simulink model "problem9"  (R2020b)
settings: Solver=ode23tb  StartTime=0.0  StopTime=1  MaxStep=Ts  RelTol=1e-3  EnableMultiTasking=on
InitFcn:
  | Ts=10e-6;
settings Model: Creator=srikanth  LastModifiedBy=Makrand Raut Dessai
settings DataIOCC: LimitDataPoints=on  SaveFormat=Array  SignalLoggingSaveFormat=ModelDataLogs  ReturnWorkspaceOutputs=off
settings OptimizationCC: ExpressionDepthLimit=2147483647  LifeSpan=inf
settings DebuggingCC: UnderspecifiedInitializationDetection=Classic  MergeDetectMultiDrivingBlocksExec=none  SolverPrmCheckMsg=warning  FcnCallInpInsideContextMsg=warning  StateNameClashWarn=warning  SFUnexpectedBacktrackingDiag=warning  SFNoUnconditionalDefaultTransitionDiag=warning  SFExecutionAtInitializationDiag=none  ArithmeticOperatorsInVariantConditions=warning
settings HardwareCC: ProdBitPerPointer=32  ProdBitPerSizeT=32  ProdBitPerPtrDiffT=32  ProdLargestAtomicFloat=None  ProdIntDivRoundTo=Undefined  ProdEndianess=Unspecified  ProdWordSize=32  ProdHWDeviceType=32-bit Generic
settings ModelReferenceCC: PropagateSignalLabelsOutOfModel=off
settings SFSimCC: SimUseLocalCustomCode=off  CustomCodeUndefinedFunction=UseInterfaceOnly
settings RTWCC: RTWUseLocalCustomCode=off
settings CodeAppCC: StateflowObjectComments=on
settings GRTTargetCC: TargetLangStandard=C89/C90 (ANSI)  CombineOutputUpdateFcns=off  GRTInterface=on
settings ConfigComp: CovMetricSettings=dw  CovSaveCumulativeToWorkspaceVar=on  CovSaveSingleToWorkspaceVar=on  CovExternalEMLEnable=off

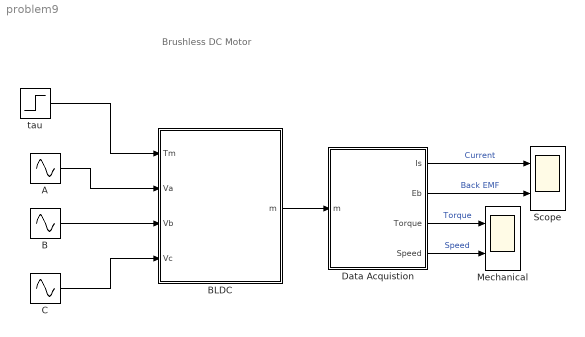
== system problem9 ==
  note: Brushless DC Motor
  A : Sin  Amplitude=220*sqrt(2)  Frequency=2*pi*50  SampleTime=Ts
  B : Sin  Amplitude=220*sqrt(2)  Frequency=2*pi*50  Phase=-2*pi/3  SampleTime=Ts
  BLDC : Subsystem  mask(Brushless DC Motor :){Rs=1.43, Ls=9.4e-3, flux=0.2158, J=1.5e-3, B=2e-3, p=4}
      mask prompts: Rs "Resistance - Rs [ohms] :"; Ls "Inductance - Ls [H] :"; flux "Flux - [wb]"; J "Rotor Inertia - J [kg-m^2]"; B "Friction Coefficient - B :"; p "No: poles of Motor :"
      mask help: Brushless DC Motor inducing trapezoidal Back EMF
      mask init:
      | trap=0.5;
      mask Display: fprintf('BLDC')
  C : Sin  Amplitude=220*sqrt(2)  Frequency=2*pi*50  Phase=2*pi/3  SampleTime=Ts
  Data Acquistion : Subsystem
  Mechanical : Scope  NumInputPorts=2
  Scope : Scope  NumInputPorts=2
  tau : Step  Time=0.5  After=10  SampleTime=0
  wires:
  BLDC/1(m) -> Data Acquistion/1(m)
  Data Acquistion/1(Is) -> Scope/1  "Current"
  Data Acquistion/2(Eb) -> Scope/2  "Back EMF"
  Data Acquistion/3(Torque) -> Mechanical/1  "Torque"
  Data Acquistion/4(Speed) -> Mechanical/2  "Speed"
  tau/1 -> BLDC/1(Tm)
  A/1 -> BLDC/2(Va)
  B/1 -> BLDC/3(Vb)
  C/1 -> BLDC/4(Vc)

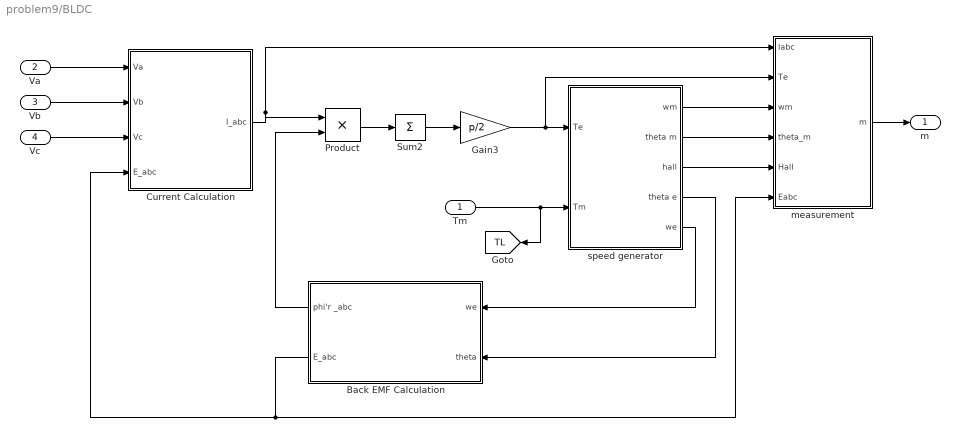
== system problem9/BLDC ==
  Tm : Inport
  Va : Inport  Port=2
  Vb : Inport  Port=3
  Vc : Inport  Port=4
  Back EMF Calculation : Subsystem
  Current Calculation : Subsystem
  Gain3 : Gain  Gain=p/2  SaturateOnIntegerOverflow=on  OutDataTypeStr=Inherit: Same as input  ParamDataTypeStr=Inherit: Same as input
  Product : Product  SaturateOnIntegerOverflow=on  OutDataTypeStr=Inherit: Same as first input
  Sum2 : Sum  Inputs=+  SaturateOnIntegerOverflow=on
  measurement : Subsystem
  speed generator : Subsystem
  m : Outport
  tag scope: TL=global
  wires:
  Vc/1 -> Current Calculation/3(Vc)
  Vb/1 -> Current Calculation/2(Vb)
  Va/1 -> Current Calculation/1(Va)
  measurement/1(m) -> m/1
  speed generator/4(theta e) -> Back EMF Calculation/2(theta)
  speed generator/3(hall) -> measurement/5(Hall)
  speed generator/2(theta m) -> measurement/4(theta_m)
  speed generator/1(wm) -> measurement/3(wm)
  Tm/1 -> [TL], speed generator/2(Tm)
  Back EMF Calculation/1(phi'r _abc) -> Product/2
  Product/1 -> Sum2/1
  Sum2/1 -> Gain3/1
  Gain3/1 -> measurement/2(Te), speed generator/1(Te)
  speed generator/5(we) -> Back EMF Calculation/1(we)
  Back EMF Calculation/2(E_abc) -> Current Calculation/4(E_abc), measurement/6(Eabc)
  Current Calculation/1(I_abc) -> Product/1, measurement/1(Iabc)

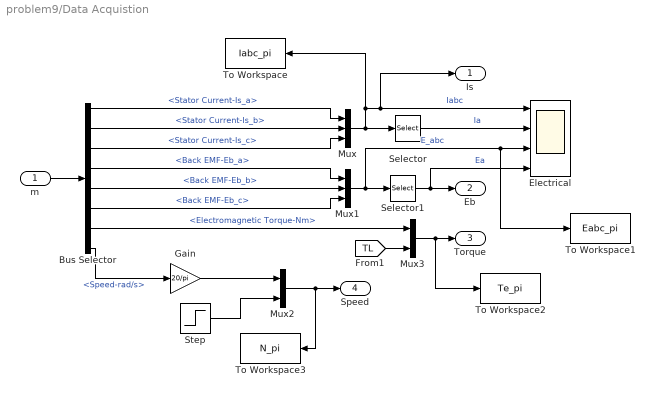
== system problem9/Data Acquistion ==
  m : Inport
  Bus Selector : BusSelector  OutputSignals=Stator Current-Is_a,Stator Current-Is_b,Stator Current-Is_c,Back EMF-Eb_a,Back EMF-Eb_b,Back EMF-Eb_c,Electromagnetic Torque-Nm,Speed-rad/s
  Electrical : Scope  NumInputPorts=4
  Gain : Gain  Gain=20/pi
  Mux : Mux  Inputs=3
  Mux1 : Mux  Inputs=3
  Mux2 : Mux  Inputs=2
  Mux3 : Mux  Inputs=2
  Selector : Selector  InputPortWidth=3  IndexOptions=Index vector (dialog)  Indices=[1 ]  OutputSizes=1
  Selector1 : Selector  InputPortWidth=3  IndexOptions=Index vector (dialog)  Indices=[1 ]  OutputSizes=1
  Step : Step  After=3000  SampleTime=0
  To Workspace : ToWorkspace  VariableName=Iabc_pi  SampleTime=Ts
  To Workspace1 : ToWorkspace  VariableName=Eabc_pi  SampleTime=Ts
  To Workspace2 : ToWorkspace  VariableName=Te_pi  SampleTime=Ts
  To Workspace3 : ToWorkspace  VariableName=N_pi  SampleTime=Ts
  Is : Outport
  Eb : Outport  Port=2
  Torque : Outport  Port=3
  Speed : Outport  Port=4
  wires:
  Mux3/1 -> To Workspace2/1, Torque/1
  [TL] -> Mux3/2
  Step/1 -> Mux2/2
  Mux2/1 -> To Workspace3/1, Speed/1
  Gain/1 -> Mux2/1
  Selector1/1 -> Electrical/4, Eb/1  "Ea"
  Selector/1 -> Electrical/2  "Ia"
  Bus Selector/8 -> Gain/1  "<Speed-rad/s>"
  Bus Selector/7 -> Mux3/1  "<Electromagnetic Torque-Nm>"
  Mux1/1 -> To Workspace1/1, Electrical/3, Selector1/1  "E_abc"
  Bus Selector/6 -> Mux1/3  "<Back EMF-Eb_c>"
  Bus Selector/5 -> Mux1/2  "<Back EMF-Eb_b>"
  Bus Selector/4 -> Mux1/1  "<Back EMF-Eb_a>"
  Mux/1 -> Is/1, Electrical/1, To Workspace/1, Selector/1  "Iabc"
  Bus Selector/3 -> Mux/3  "<Stator Current-Is_c>"
  Bus Selector/2 -> Mux/2  "<Stator Current-Is_b>"
  Bus Selector/1 -> Mux/1  "<Stator Current-Is_a>"
  m/1 -> Bus Selector/1

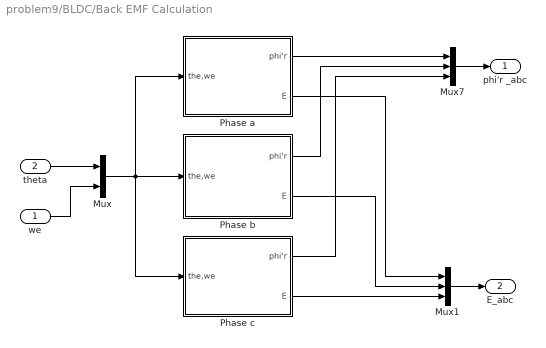
== system problem9/BLDC/Back EMF Calculation ==
  we : Inport
  theta : Inport  Port=2
  Mux : Mux  Inputs=2
  Mux1 : Mux  Inputs=3
  Mux7 : Mux  Inputs=3
  Phase a : Subsystem
  Phase b : Subsystem
  Phase c : Subsystem
  phi'r _abc : Outport
  E_abc : Outport  Port=2
  wires:
  Mux1/1 -> E_abc/1
  Phase c/2(E) -> Mux1/3
  Phase b/2(E) -> Mux1/2
  Phase a/2(E) -> Mux1/1
  we/1 -> Mux/2
  theta/1 -> Mux/1
  Mux/1 -> Phase c/1(the,we), Phase b/1(the,we), Phase a/1(the,we)
  Phase a/1(phi'r) -> Mux7/1
  Phase b/1(phi'r) -> Mux7/2
  Phase c/1(phi'r) -> Mux7/3
  Mux7/1 -> phi'r _abc/1

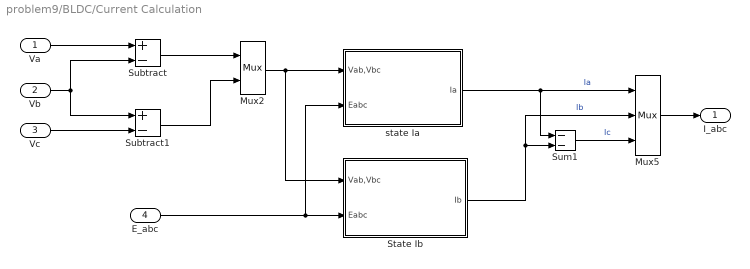
== system problem9/BLDC/Current Calculation ==
  Va : Inport
  Vb : Inport  Port=2
  Vc : Inport  Port=3
  E_abc : Inport  Port=4
  Mux2 : Mux  Inputs=2
      settings: DisplayOption=signals
  Mux5 : Mux  Inputs=3
      settings: DisplayOption=signals
  State Ib : Subsystem
  Subtract : Sum  Inputs=+-
  Subtract1 : Sum  Inputs=+-
  Sum1 : Sum  Inputs=--  SaturateOnIntegerOverflow=on
  state Ia : Subsystem
  I_abc : Outport
  wires:
  State Ib/1(Ib) -> Sum1/2, Mux5/2  "Ib"
  Subtract1/1 -> Mux2/2
  Subtract/1 -> Mux2/1
  Vc/1 -> Subtract1/2
  Vb/1 -> Subtract1/1, Subtract/2
  Va/1 -> Subtract/1
  state Ia/1(Ia) -> Mux5/1, Sum1/1  "Ia"
  Sum1/1 -> Mux5/3  "Ic"
  Mux5/1 -> I_abc/1
  Mux2/1 -> State Ib/1(Vab,Vbc), state Ia/1(Vab,Vbc)
  E_abc/1 -> State Ib/2(Eabc), state Ia/2(Eabc)

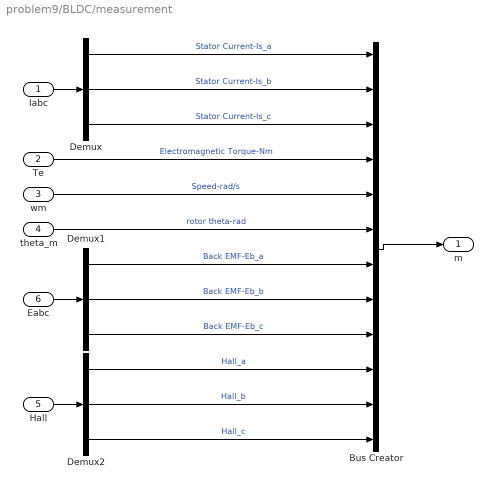
== system problem9/BLDC/measurement ==
  Iabc : Inport
  Te : Inport  Port=2
  wm : Inport  Port=3
  theta_m : Inport  Port=4
  Hall : Inport  Port=5
  Eabc : Inport  Port=6
  Bus Creator : BusCreator  Inputs=12
  Demux : Demux  Outputs=3
  Demux1 : Demux  Outputs=3
  Demux2 : Demux  Outputs=3
  m : Outport
  wires:
  theta_m/1 -> Bus Creator/6  "rotor theta-rad"
  Demux2/3 -> Bus Creator/12  "Hall_c"
  Demux2/2 -> Bus Creator/11  "Hall_b"
  Demux2/1 -> Bus Creator/10  "Hall_a"
  Hall/1 -> Demux2/1
  Demux1/3 -> Bus Creator/9  "Back EMF-Eb_c"
  Demux1/2 -> Bus Creator/8  "Back EMF-Eb_b"
  Demux1/1 -> Bus Creator/7  "Back EMF-Eb_a"
  Eabc/1 -> Demux1/1
  Demux/2 -> Bus Creator/2  "Stator Current-Is_b"
  Bus Creator/1 -> m/1
  wm/1 -> Bus Creator/5  "Speed-rad/s"
  Te/1 -> Bus Creator/4  "Electromagnetic Torque-Nm"
  Demux/3 -> Bus Creator/3  "Stator Current-Is_c"
  Demux/1 -> Bus Creator/1  "Stator Current-Is_a"
  Iabc/1 -> Demux/1

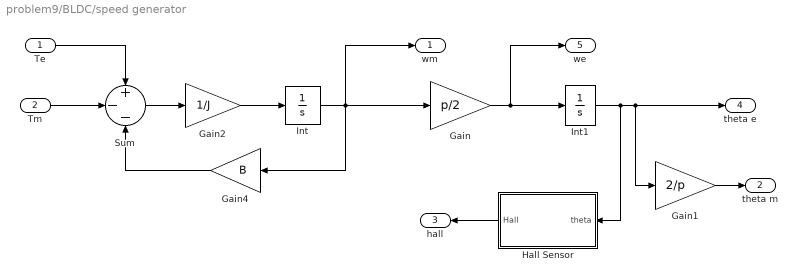
== system problem9/BLDC/speed generator ==
  Te : Inport
  Tm : Inport  Port=2
  Gain : Gain  Gain=p/2  SaturateOnIntegerOverflow=on  OutDataTypeStr=Inherit: Same as input  ParamDataTypeStr=Inherit: Same as input
  Gain1 : Gain  Gain=2/p  SaturateOnIntegerOverflow=on  OutDataTypeStr=Inherit: Same as input  ParamDataTypeStr=Inherit: Same as input
  Gain2 : Gain  Gain=1/J  SaturateOnIntegerOverflow=on  OutDataTypeStr=Inherit: Same as input  ParamDataTypeStr=Inherit: Same as input
  Gain4 : Gain  Gain=B  SaturateOnIntegerOverflow=on  OutDataTypeStr=Inherit: Same as input  ParamDataTypeStr=Inherit: Same as input
  Hall Sensor : Subsystem
  Int : Integrator
  Int1 : Integrator
  Sum : Sum  Inputs=+--  InputSameDT=on  SaturateOnIntegerOverflow=on  OutDataTypeStr=Inherit: Same as first input
  wm : Outport
  theta m : Outport  Port=2
  hall : Outport  Port=3
  theta e : Outport  Port=4
  we : Outport  Port=5
  wires:
  Gain1/1 -> theta m/1
  Hall Sensor/1(Hall) -> hall/1
  Te/1 -> Sum/1
  Tm/1 -> Sum/2
  Gain4/1 -> Sum/3
  Sum/1 -> Gain2/1
  Gain2/1 -> Int/1
  Int/1 -> wm/1, Gain4/1, Gain/1
  Gain/1 -> we/1, Int1/1
  Int1/1 -> Gain1/1, theta e/1, Hall Sensor/1(theta)

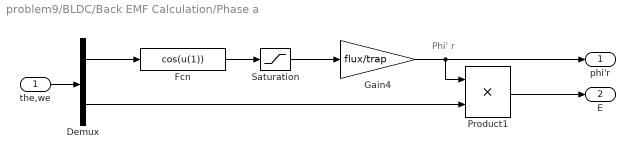
== system problem9/BLDC/Back EMF Calculation/Phase a ==
  note: Phi' r
  the,we : Inport
  Demux : Demux  Outputs=2
      settings: DisplayOption=none
  Fcn : Fcn  Expr=cos(u(1))
  Gain4 : Gain  Gain=flux/trap  SaturateOnIntegerOverflow=on  OutDataTypeStr=Inherit: Same as input  ParamDataTypeStr=Inherit: Same as input
  Product1 : Product  SaturateOnIntegerOverflow=on  OutDataTypeStr=Inherit: Same as first input
  Saturation : Saturate  UpperLimit=trap  LowerLimit=-trap
  phi'r : Outport
  E : Outport  Port=2
  wires:
  Fcn/1 -> Saturation/1
  Saturation/1 -> Gain4/1
  Demux/1 -> Fcn/1
  Demux/2 -> Product1/2
  the,we/1 -> Demux/1
  Product1/1 -> E/1
  Gain4/1 -> phi'r/1, Product1/1

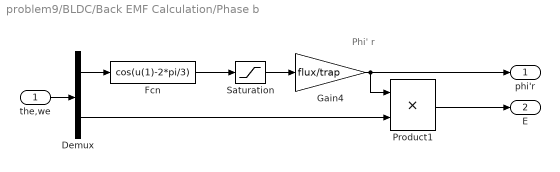
== system problem9/BLDC/Back EMF Calculation/Phase b ==
  note: Phi' r
  the,we : Inport
  Demux : Demux  Outputs=2
      settings: DisplayOption=none
  Fcn : Fcn  Expr=cos(u(1)-2*pi/3)
  Gain4 : Gain  Gain=flux/trap  SaturateOnIntegerOverflow=on  OutDataTypeStr=Inherit: Same as input  ParamDataTypeStr=Inherit: Same as input
  Product1 : Product  SaturateOnIntegerOverflow=on  OutDataTypeStr=Inherit: Same as first input
  Saturation : Saturate  UpperLimit=trap  LowerLimit=-trap
  phi'r : Outport
  E : Outport  Port=2
  wires:
  Fcn/1 -> Saturation/1
  Saturation/1 -> Gain4/1
  Gain4/1 -> Product1/1, phi'r/1
  Product1/1 -> E/1
  the,we/1 -> Demux/1
  Demux/2 -> Product1/2
  Demux/1 -> Fcn/1

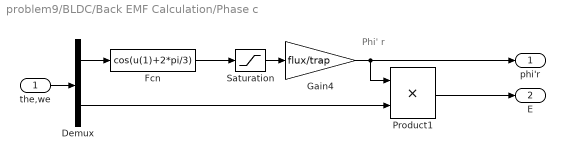
== system problem9/BLDC/Back EMF Calculation/Phase c ==
  note: Phi' r
  the,we : Inport
  Demux : Demux  Outputs=2
      settings: DisplayOption=none
  Fcn : Fcn  Expr=cos(u(1)+2*pi/3)
  Gain4 : Gain  Gain=flux/trap  SaturateOnIntegerOverflow=on  OutDataTypeStr=Inherit: Same as input  ParamDataTypeStr=Inherit: Same as input
  Product1 : Product  SaturateOnIntegerOverflow=on  OutDataTypeStr=Inherit: Same as first input
  Saturation : Saturate  UpperLimit=trap  LowerLimit=-trap
  phi'r : Outport
  E : Outport  Port=2
  wires:
  Fcn/1 -> Saturation/1
  Saturation/1 -> Gain4/1
  Demux/1 -> Fcn/1
  Demux/2 -> Product1/2
  the,we/1 -> Demux/1
  Product1/1 -> E/1
  Gain4/1 -> phi'r/1, Product1/1

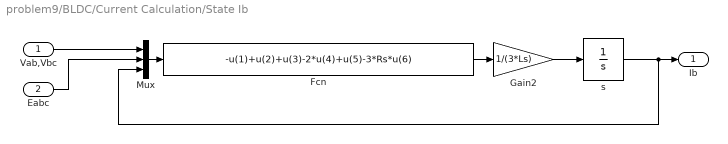
== system problem9/BLDC/Current Calculation/State Ib ==
  Vab,Vbc : Inport
  Eabc : Inport  Port=2
  Fcn : Fcn  Expr=-u(1)+u(2)+u(3)-2*u(4)+u(5)-3*Rs*u(6)
  Gain2 : Gain  Gain=1/(3*Ls)  SaturateOnIntegerOverflow=on  OutDataTypeStr=Inherit: Same as input  ParamDataTypeStr=Inherit: Same as input
  Mux : Mux  Inputs=3
  "s " : Integrator
  Ib : Outport
  wires:
  "s "/1 -> Ib/1, Mux/3
  Fcn/1 -> Gain2/1
  Mux/1 -> Fcn/1
  Eabc/1 -> Mux/2
  Vab,Vbc/1 -> Mux/1
  Gain2/1 -> "s "/1

== system problem9/BLDC/Current Calculation/state Ia ==
  Vab,Vbc : Inport
  Eabc : Inport  Port=2
  Fcn : Fcn  Expr=2*u(1)+u(2)-2*u(3)+u(4)+u(5)-3*Rs*u(6)
  Gain2 : Gain  Gain=1/(3*Ls)  SaturateOnIntegerOverflow=on  OutDataTypeStr=Inherit: Same as input  ParamDataTypeStr=Inherit: Same as input
  Mux : Mux  Inputs=3
  "s " : Integrator
  Ia : Outport
  wires:
  Gain2/1 -> "s "/1
  Vab,Vbc/1 -> Mux/1
  Eabc/1 -> Mux/2
  Mux/1 -> Fcn/1
  Fcn/1 -> Gain2/1
  "s "/1 -> Ia/1, Mux/3

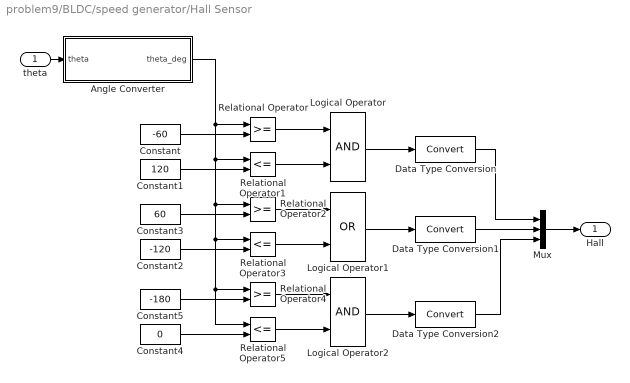
== system problem9/BLDC/speed generator/Hall Sensor ==
  theta : Inport
  Angle Converter : Subsystem
  Constant : Constant  Value=-60
  Constant1 : Constant  Value=120
  Constant2 : Constant  Value=-120
  Constant3 : Constant  Value=60
  Constant4 : Constant  Value=0
  Constant5 : Constant  Value=-180
  Data Type Conversion : DataTypeConversion
  Data Type Conversion1 : DataTypeConversion
  Data Type Conversion2 : DataTypeConversion
  Logical Operator : Logic  AllPortsSameDT=off  OutDataTypeStr=boolean
  Logical Operator1 : Logic  Operator=OR  AllPortsSameDT=off  OutDataTypeStr=boolean
  Logical Operator2 : Logic  AllPortsSameDT=off  OutDataTypeStr=boolean
  Mux : Mux  Inputs=3
  Relational Operator : RelationalOperator  OutDataTypeStr=boolean  RndMeth=Nearest
  Relational Operator1 : RelationalOperator  Operator=<=  OutDataTypeStr=boolean  RndMeth=Nearest
  Relational Operator2 : RelationalOperator  OutDataTypeStr=boolean  RndMeth=Nearest
  Relational Operator3 : RelationalOperator  Operator=<=  OutDataTypeStr=boolean  RndMeth=Nearest
  Relational Operator4 : RelationalOperator  OutDataTypeStr=boolean  RndMeth=Nearest
  Relational Operator5 : RelationalOperator  Operator=<=  OutDataTypeStr=boolean  RndMeth=Nearest
  Hall : Outport
  wires:
  Mux/1 -> Hall/1
  Data Type Conversion2/1 -> Mux/3
  Data Type Conversion1/1 -> Mux/2
  Data Type Conversion/1 -> Mux/1
  Logical Operator/1 -> Data Type Conversion/1
  Logical Operator1/1 -> Data Type Conversion1/1
  Logical Operator2/1 -> Data Type Conversion2/1
  Relational Operator5/1 -> Logical Operator2/2
  Relational Operator4/1 -> Logical Operator2/1
  Relational Operator3/1 -> Logical Operator1/2
  Relational Operator2/1 -> Logical Operator1/1
  Relational Operator1/1 -> Logical Operator/2
  Relational Operator/1 -> Logical Operator/1
  Constant4/1 -> Relational Operator5/2
  Constant5/1 -> Relational Operator4/2
  Constant2/1 -> Relational Operator3/2
  Constant3/1 -> Relational Operator2/2
  Constant1/1 -> Relational Operator1/2
  Constant/1 -> Relational Operator/2
  Angle Converter/1(theta_deg) -> Relational Operator5/1, Relational Operator4/1, Relational Operator3/1, Relational Operator2/1, Relational Operator1/1, Relational Operator/1
  theta/1 -> Angle Converter/1(theta)

== system problem9/BLDC/speed generator/Hall Sensor/Angle Converter ==
  theta : Inport
  Trigonometric Function : Trigonometry
  Trigonometric Function1 : Trigonometry  Operator=cos
  Trigonometric Function2 : Trigonometry  Operator=atan2
  rad2deg : Gain  Gain=180/pi
  theta_deg : Outport
  wires:
  rad2deg/1 -> theta_deg/1
  theta/1 -> Trigonometric Function1/1, Trigonometric Function/1
  Trigonometric Function1/1 -> Trigonometric Function2/2
  Trigonometric Function/1 -> Trigonometric Function2/1
  Trigonometric Function2/1 -> rad2deg/1
